simulink model "Model1_3_ZVD"  (R2021a)
settings: Solver=VariableStepAuto  StartTime=0.0  StopTime=20  RelTol=1e-3
InitFcn:
  | ml=2;
  | 
  | mc=0.5;
  | M2=0.5;
  | 
  | mt=5;
  | g=9.81;
  | l_ref=0.1;
  | l_ini=1;
  | l=l_ini;
  | x_ref=1;
  | n1=5;n2=1;
  | 
  | %ADRC' s parameter caculation
  | %b0 = (ml+mc)/(mc*ml +mc*mt+ml*mt); %Hieu
  | b0=(ml+mc)/(mt*mc+2*ml*mc+mt*ml+ml^2+mc^2); %Enhanced-coupling
  | k_ESO = 100;
  | T_set  = 6;
  | 
  | s_cl = -5.85/T_set;
  | Kp   = s_cl^2;
  | Kd   = -2*s_cl;
  | 
  | s_ESO = k_ESO*s_cl;
  | l1        = -3*s_ESO;
  | l2        = 3*( s_ESO)^2;
  | l3        = -(s_ESO)^3;
  | 
  | %b1 = (mt+mc)/(mc*ml +mc*mt+ml*mt);
  | b1=1/(ml+mc);
  | k_ESO1 =100;
  | T_set1  = 3;
  | s_cl1 = -5.85/T_set1;
  | Kp1   = s_cl1^2;
  | Kd1   = -2*s_cl1;
  | 
  | s_ESO1 = k_ESO1*s_cl1;
  | l11        = -3*s_ESO1;
  | l21        = 3*( s_ESO1)^2;
  | l31        = -(s_ESO1)^3;
  | 
  | 
  | L1=l_ini;
  | %L2=0.5;
  | L2=0.1;
  | m1=2;
  | m2=mc;
  | m=5;
  | %Bo input shaping
  | alpha = (1/L1 + 1/L2)*(m1+M2)/m1;
  | beta = (((m1+M2)/m1)^2)*((1/L1 + 1/L2)^2) - 4*(m1+M2)/(m1*L1*L2);
  | w1 = sqrt(g*(alpha - sqrt(beta))/2);
  | w2 = sqrt(g*(alpha + sqrt(beta))/2);
  | damping_ratio = 0;
  | wd1 = w1*sqrt(1-damping_ratio^2);
  | wd2 = w2*sqrt(1-damping_ratio^2);
  | k = exp(damping_ratio*pi/sqrt(1-damping_ratio^2));
  | 
  | %ZVD1
  | t1_ZVD_1=pi/wd1;
  | ... (+27 lines)
values from neighbouring files (symbols this model uses):
  particle = repmat(empty_particle, nPop, 1)    [PSO16_12.m]    (also in PSO_ZVD.m)
undefined symbols (not defined in the file or in its folder): E1_tt, E2_tt, E3_tt, i, li, xi
libraries: neural x66, simulink_extras x4, simulink x2
(part 12 of 20)

== matlab function Model1_3_ZVD/non linear model/con lắc đôi2/MATLAB Function ==
  data: z1 input; z2 input; z3 input; z4 input; z5 input; z6 input; z7 input; z8 input; d1z1 output; d1z2 output; d1z3 output; d1z4 output; d1z5 output; d1z6 output; d1z7 output; d1z8 output; ux input; ul input
function [d1z1,d1z2,d1z3,d1z4,d1z5,d1z6,d1z7,d1z8] = fcn(z1,z2, z3, z4, z5, z6, z7, z8, ux, ul)

m=20; m1=5; m2=1; l2= 0.2; g= 9.8;

d1z1=z2;
d1z2 =(m1*ul*sin(z5) - m2*ux - m1*ux + m2*ul*sin(z5) + m2*ux*cos(z5 - z7)^2 + m2*ux*sin(z5 - z7)^2 - m2*ul*sin(z5 - z7)*cos(z7) - g*m2^2*cos(z7)*sin(z7) - l2*m2^2*z8^2*sin(z7) - m2*ul*cos(z5 - z7)^2*sin(z5) + g*m2^2*cos(z5 - z7)*sin(z5 - z7)*cos(z5)^2 - g*m2^2*cos(z5 - z7)*sin(z5 - z7)*sin(z5)^2 + m2*ul*cos(z5 - z7)*sin(z5 - z7)*cos(z5) - g*m1*m2*cos(z7)*sin(z7) - l2*m1*m2*z8^2*sin(z7) + g*m2^2*cos(z5 - z7)*cos(z5)*sin(z7) + g*m2^2*cos(z5 - z7)*cos(z7)*sin(z5) - g*m2^2*sin(z5 - z7)*cos(z5)*cos(z7) + l2*m2^2*z8^2*cos(z5 - z7)*sin(z5) - l2*m2^2*z8^2*sin(z5 - z7)*cos(z5) + g*m2^2*sin(z5 - z7)*sin(z5)*sin(z7) - g*m2^2*cos(z5 - z7)^2*cos(z5)*sin(z5) - l2*m2^2*z8^2*cos(z5 - z7)^3*sin(z5) + l2*m2^2*z8^2*sin(z5 - z7)^3*cos(z5) + l2*m2^2*z8^2*cos(z5 - z7)^2*sin(z7) + g*m2^2*sin(z5 - z7)^2*cos(z5)*sin(z5) + l2*m2^2*z8^2*sin(z5 - z7)^2*sin(z7) + g*m1*m2*cos(z5 - z7)*sin(z5 - z7)*cos(z5)^2 - g*m1*m2*cos(z5 - z7)*sin(z5 - z7)*sin(z5)^2 + g*m1*m2*cos(z5 - z7)*cos(z5)*sin(z7) + g*m1*m2*cos(z5 - z7)*cos(z7)*sin(z5) - g*m1*m2*sin(z5 - z7)*cos(z5)*cos(z7) + l2*m1*m2*z8^2*cos(z5 - z7)*sin(z5) - l2*m1*m2*z8^2*sin(z5 - z7)*cos(z5) + g*m1*m2*sin(z5 - z7)*sin(z5)*sin(z7) - g*m1*m2*cos(z5 - z7)^2*cos(z5)*sin(z5) + l2*m2^2*z8^2*cos(z5 - z7)^2*sin(z5 - z7)*cos(z5) + g*m1*m2*sin(z5 - z7)^2*cos(z5)*sin(z5) - l2*m2^2*z8^2*cos(z5 - z7)*sin(z5 - z7)^2*sin(z5))/(m1^2*cos(z5)^2 - m*m2 - 2*m1*m2 - m*m1 + m2^2*cos(z5)^2 + m2^2*cos(z7)^2 + m1^2*sin(z5)^2 + m2^2*sin(z5)^2 + m2^2*cos(z5 - z7)^2 + m2^2*sin(z5 - z7)^2 - m1^2 - m2^2 + 2*m1*m2*cos(z5)^2 + m1*m2*cos(z7)^2 + 2*m1*m2*sin(z5)^2 + m*m2*cos(z5 - z7)^2 + m1*m2*cos(z5 - z7)^2 + m*m2*sin(z5 - z7)^2 + m1*m2*sin(z5 - z7)^2 - m2^2*cos(z5 - z7)^2*sin(z5)^2 - m2^2*sin(z5 - z7)^2*cos(z5)^2 - 2*m2^2*sin(z5 - z7)*cos(z7)*sin(z5) - m1*m2*cos(z5 - z7)^2*sin(z5)^2 - m1*m2*sin(z5 - z7)^2*cos(z5)^2 - 2*m2^2*cos(z5 - z7)*cos(z5)*cos(z7) - 2*m1*m2*cos(z5 - z7)*cos(z5)*cos(z7) - 2*m1*m2*sin(z5 - z7)*cos(z7)*sin(z5) + 2*m2^2*cos(z5 - z7)*sin(z5 - z7)*cos(z5)*sin(z5) + 2*m1*m2*cos(z5 - z7)*sin(z5 - z7)*cos(z5)*sin(z5));
d1z3=z4; 
d1z4 =(m2^2*ul*cos(z5 - z7)^2 - m2^2*ul - m1^2*ul - g*m1^3*cos(z5) - g*m2^3*cos(z5) - m1^3*z3*z6^2 - m2^3*z3*z6^2 + m1^2*ux*sin(z5) + m2^2*ux*sin(z5) - m*m1*ul - m*m2*ul - 2*m1*m2*ul + g*m1^3*cos(z5)^3 + g*m2^3*cos(z5)^3 + m1^2*ul*cos(z5)^2 + m2^2*ul*cos(z5)^2 + m2^2*ul*cos(z7)^2 - m2^2*ux*cos(z5 - z7)^2*sin(z5) + m2^3*z3*z6^2*sin(z5 - z7)^2 + m*m2*ul*cos(z5 - z7)^2 + m1*m2*ul*cos(z5 - z7)^2 + 3*g*m1*m2^2*cos(z5)^3 + 3*g*m1^2*m2*cos(z5)^3 - l2*m2^3*z8^2*cos(z5 - z7) + 2*m1*m2*ux*sin(z5) - m2^2*ux*sin(z5 - z7)*cos(z7) - g*m2^3*sin(z5 - z7)*sin(z7) + g*m2^3*cos(z5)*cos(z7)^2 + m1^3*z3*z6^2*cos(z5)^2 + m2^3*z3*z6^2*cos(z5)^2 + m2^3*z3*z6^2*cos(z7)^2 + g*m1^3*cos(z5)*sin(z5)^2 + g*m2^3*cos(z5)*sin(z5)^2 + m1^3*z3*z6^2*sin(z5)^2 + m2^3*z3*z6^2*sin(z5)^2 - g*m*m1^2*cos(z5) - g*m*m2^2*cos(z5) - 3*g*m1*m2^2*cos(z5) - 3*g*m1^2*m2*cos(z5) + g*m2^3*cos(z5 - z7)^2*cos(z5) + l2*m2^3*z8^2*cos(z5 - z7)^3 + 2*m1*m2*ul*cos(z5)^2 + m1*m2*ul*cos(z7)^2 - m*m1^2*z3*z6^2 - m*m2^2*z3*z6^2 - 3*m1*m2^2*z3*z6^2 - 3*m1^2*m2*z3*z6^2 + m2^3*z3*z6^2*cos(z5 - z7)^2 + l2*m2^3*z8^2*cos(z5 - z7)*sin(z5 - z7)^2 - m1*m2*ux*cos(z5 - z7)^2*sin(z5) - g*m*m2^2*sin(z5 - z7)*sin(z7) - 2*g*m1*m2^2*sin(z5 - z7)*sin(z7) - g*m1^2*m2*sin(z5 - z7)*sin(z7) + 2*g*m1*m2^2*cos(z5)*cos(z7)^2 + g*m1^2*m2*cos(z5)*cos(z7)^2 + 3*m1*m2^2*z3*z6^2*cos(z5)^2 + 3*m1^2*m2*z3*z6^2*cos(z5)^2 + 2*m1*m2^2*z3*z6^2*cos(z7)^2 + m1^2*m2*z3*z6^2*cos(z7)^2 + 3*g*m1*m2^2*cos(z5)*sin(z5)^2 + 3*g*m1^2*m2*cos(z5)*sin(z5)^2 + 3*m1*m2^2*z3*z6^2*sin(z5)^2 + 3*m1^2*m2*z3*z6^2*sin(z5)^2 - m2^3*z3*z6^2*cos(z5 - z7)^2*sin(z5)^2 - m2^3*z3*z6^2*sin(z5 - z7)^2*cos(z5)^2 + g*m2^3*cos(z7)*sin(z5)*sin(z7) + l2*m2^3*z8^2*sin(z5)*sin(z7) + g*m*m2^2*cos(z5 - z7)^2*cos(z5) + 2*g*m1*m2^2*cos(z5 - z7)^2*cos(z5) + g*m1^2*m2*cos(z5 - z7)^2*cos(z5) + l2*m*m2^2*z8^2*cos(z5 - z7)^3 + l2*m1*m2^2*z8^2*cos(z5 - z7)^3 + m*m2^2*z3*z6^2*cos(z5 - z7)^2 + 2*m1*m2^2*z3*z6^2*cos(z5 - z7)^2 + m1^2*m2*z3*z6^2*cos(z5 - z7)^2 + m*m2^2*z3*z6^2*sin(z5 - z7)^2 + 2*m1*m2^2*z3*z6^2*sin(z5 - z7)^2 + m1^2*m2*z3*z6^2*sin(z5 - z7)^2 - 2*m2^2*ul*cos(z5 - z7)*cos(z5)*cos(z7) - m1*m2*ux*sin(z5 - z7)*cos(z7) + m2^2*ux*cos(z5 - z7)*sin(z5 - z7)*cos(z5) + g*m2^3*cos(z5 - z7)*sin(z5 - z7)*sin(z5) - 2*g*m2^3*cos(z5 - z7)*cos(z5)^2*cos(z7) + l2*m2^3*z8^2*cos(z5 - z7)*cos(z5)^2 + l2*m2^3*z8^2*cos(z5 - z7)*cos(z7)^2 - g*m2^3*cos(z5 - z7)*cos(z7)*sin(z5)^2 + g*m2^3*sin(z5 - z7)*cos(z5)^2*sin(z7) - 2*g*m*m1*m2*cos(z5) - l2*m*m2^2*z8^2*cos(z5 - z7) - 2*l2*m1*m2^2*z8^2*cos(z5 - z7) - l2*m1^2*m2*z8^2*cos(z5 - z7) - 2*m*m1*m2*z3*z6^2 - l2*m*m1*m2*z8^2*cos(z5 - z7) - g*m*m1*m2*sin(z5 - z7)*sin(z7) + g*m*m2^2*cos(z5 - z7)*sin(z5 - z7)*sin(z5) + 2*g*m1*m2^2*cos(z5 - z7)*sin(z5 - z7)*sin(z5) + g*m1^2*m2*cos(z5 - z7)*sin(z5 - z7)*sin(z5) - 4*g*m1*m2^2*cos(z5 - z7)*cos(z5)^2*cos(z7) - 2*g*m1^2*m2*cos(z5 - z7)*cos(z5)^2*cos(z7) + 2*l2*m1*m2^2*z8^2*cos(z5 - z7)*cos(z5)^2 + l2*m1^2*m2*z8^2*cos(z5 - z7)*cos(z5)^2 + l2*m1*m2^2*z8^2*cos(z5 - z7)*cos(z7)^2 - 2*g*m1*m2^2*cos(z5 - z7)*cos(z7)*sin(z5)^2 - g*m1^2*m2*cos(z5 - z7)*cos(z7)*sin(z5)^2 + 2*g*m1*m2^2*sin(z5 - z7)*cos(z5)^2*sin(z7) + g*m1^2*m2*sin(z5 - z7)*cos(z5)^2*sin(z7) - 2*m2^3*z3*z6^2*cos(z5 - z7)*cos(z5)*cos(z7) + g*m*m1*m2*cos(z5 - z7)^2*cos(z5) - g*m2^3*cos(z5 - z7)*cos(z5)*sin(z5)*sin(z7) - g*m2^3*sin(z5 - z7)*cos(z5)*cos(z7)*sin(z5) + l2*m2^3*z8^2*sin(z5 - z7)*cos(z5)*sin(z5) - l2*m2^3*z8^2*sin(z5 - z7)*cos(z7)*sin(z7) + m*m1*m2*z3*z6^2*cos(z5 - z7)^2 - 2*m2^3*z3*z6^2*sin(z5 - z7)*cos(z7)*sin(z5) + l2*m*m2^2*z8^2*cos(z5 - z7)*sin(z5 - z7)^2 + l2*m1*m2^2*z8^2*cos(z5 - z7)*sin(z5 - z7)^2 + m*m1*m2*z3*z6^2*sin(z5 - z7)^2 - 2*m1*m2*ul*cos(z5 - z7)*cos(z5)*cos(z7) - 2*l2*m2^3*z8^2*cos(z5 - z7)^2*cos(z5)*cos(z7) - 2*m1*m2^2*z3*z6^2*cos(z5 - z7)^2*sin(z5)^2 - 2*m1*m2^2*z3*z6^2*sin(z5 - z7)^2*cos(z5)^2 - m1^2*m2*z3*z6^2*cos(z5 - z7)^2*sin(z5)^2 - m1^2*m2*z3*z6^2*sin(z5 - z7)^2*cos(z5)^2 - l2*m2^3*z8^2*sin(z5 - z7)^2*cos(z5)*cos(z7) + 2*g*m1*m2^2*cos(z7)*sin(z5)*sin(z7) + g*m1^2*m2*cos(z7)*sin(z5)*sin(z7) + 2*l2*m1*m2^2*z8^2*sin(z5)*sin(z7) + l2*m1^2*m2*z8^2*sin(z5)*sin(z7) - l2*m2^3*z8^2*cos(z5 - z7)^2*sin(z5)*sin(z7) + m1*m2*ux*cos(z5 - z7)*sin(z5 - z7)*cos(z5) - 2*l2*m1*m2^2*z8^2*cos(z5 - z7)^2*cos(z5)*cos(z7) - l2*m1*m2^2*z8^2*sin(z5 - z7)^2*cos(z5)*cos(z7) - l2*m1*m2^2*z8^2*cos(z5 - z7)^2*sin(z5)*sin(z7) + g*m*m1*m2*cos(z5 - z7)*sin(z5 - z7)*sin(z5) + l2*m2^3*z8^2*cos(z5 - z7)*sin(z5 - z7)*cos(z5)*sin(z7) - l2*m2^3*z8^2*cos(z5 - z7)*sin(z5 - z7)*cos(z7)*sin(z5) + 2*m2^3*z3*z6^2*cos(z5 - z7)*sin(z5 - z7)*cos(z5)*sin(z5) - 4*m1*m2^2*z3*z6^2*cos(z5 - z7)*cos(z5)*cos(z7) - 2*m1^2*m2*z3*z6^2*cos(z5 - z7)*cos(z5)*cos(z7) - 2*g*m1*m2^2*cos(z5 - z7)*cos(z5)*sin(z5)*sin(z7) - 2*g*m1*m2^2*sin(z5 - z7)*cos(z5)*cos(z7)*sin(z5) - g*m1^2*m2*cos(z5 - z7)*cos(z5)*sin(z5)*sin(z7) - g*m1^2*m2*sin(z5 - z7)*cos(z5)*cos(z7)*sin(z5) + 2*l2*m1*m2^2*z8^2*sin(z5 - z7)*cos(z5)*sin(z5) + l2*m1^2*m2*z8^2*sin(z5 - z7)*cos(z5)*sin(z5) - l2*m1*m2^2*z8^2*sin(z5 - z7)*cos(z7)*sin(z7) - 4*m1*m2^2*z3*z6^2*sin(z5 - z7)*cos(z7)*sin(z5) - 2*m1^2*m2*z3*z6^2*sin(z5 - z7)*cos(z7)*sin(z5) + l2*m1*m2^2*z8^2*cos(z5 - z7)*sin(z5 - z7)*cos(z5)*sin(z7) - l2*m1*m2^2*z8^2*cos(z5 - z7)*sin(z5 - z7)*cos(z7)*sin(z5) + 4*m1*m2^2*z3*z6^2*cos(z5 - z7)*sin(z5 - z7)*cos(z5)*sin(z5) + 2*m1^2*m2*z3*z6^2*cos(z5 - z7)*sin(z5 - z7)*cos(z5)*sin(z5))/((m1 + m2)*(m1^2*cos(z5)^2 - m*m2 - 2*m1*m2 - m*m1 + m2^2*cos(z5)^2 + m2^2*cos(z7)^2 + m1^2*sin(z5)^2 + m2^2*sin(z5)^2 + m2^2*cos(z5 - z7)^2 + m2^2*sin(z5 - z7)^2 - m1^2 - m2^2 + 2*m1*m2*cos(z5)^2 + m1*m2*cos(z7)^2 + 2*m1*m2*sin(z5)^2 + m*m2*cos(z5 - z7)^2 + m1*m2*cos(z5 - z7)^2 + m*m2*sin(z5 - z7)^2 + m1*m2*sin(z5 - z7)^2 - m2^2*cos(z5 - z7)^2*sin(z5)^2 - m2^2*sin(z5 - z7)^2*cos(z5)^2 - 2*m2^2*sin(z5 - z7)*cos(z7)*sin(z5) - m1*m2*cos(z5 - z7)^2*sin(z5)^2 - m1*m2*sin(z5 - z7)^2*cos(z5)^2 - 2*m2^2*cos(z5 - z7)*cos(z5)*cos(z7) - 2*m1*m2*cos(z5 - z7)*cos(z5)*cos(z7) - 2*m1*m2*sin(z5 - z7)*cos(z7)*sin(z5) + 2*m2^2*cos(z5 - z7)*sin(z5 - z7)*cos(z5)*sin(z5) + 2*m1*m2*cos(z5 - z7)*sin(z5 - z7)*cos(z5)*sin(z5)));
d1z5=z6; 
d1z6 =-(g*m1^3*sin(z5)^3 - 2*m2^3*z4*z6 - m1^2*ux*cos(z5) - m2^2*ux*cos(z5) - g*m1^3*sin(z5) - g*m2^3*sin(z5) - 2*m1^3*z4*z6 + g*m2^3*sin(z5)^3 + m2^2*ux*sin(z5 - z7)^2*cos(z5) + g*m2^3*sin(z5 - z7)^2*sin(z5) + 3*g*m1*m2^2*sin(z5)^3 + 3*g*m1^2*m2*sin(z5)^3 + 2*m1^3*z4*z6*cos(z5)^2 + 2*m2^3*z4*z6*cos(z5)^2 + 2*m2^3*z4*z6*cos(z7)^2 + m1^2*ul*cos(z5)*sin(z5) + m2^2*ul*cos(z5)*sin(z5) + 2*m1^3*z4*z6*sin(z5)^2 + 2*m2^3*z4*z6*sin(z5)^2 - 2*m1*m2*ux*cos(z5) - 2*m*m1^2*z4*z6 - 2*m*m2^2*z4*z6 - 6*m1*m2^2*z4*z6 - 6*m1^2*m2*z4*z6 + m2^2*ux*cos(z5 - z7)*cos(z7) + 2*m2^3*z4*z6*cos(z5 - z7)^2 + g*m2^3*cos(z5 - z7)*sin(z7) - l2*m2^3*z8^2*sin(z5 - z7) + 2*m2^3*z4*z6*sin(z5 - z7)^2 + g*m1^3*cos(z5)^2*sin(z5) + g*m2^3*cos(z5)^2*sin(z5) + g*m2^3*cos(z7)^2*sin(z5) + m2^2*ul*cos(z5 - z7)*sin(z5 - z7) - g*m*m1^2*sin(z5) - g*m*m2^2*sin(z5) - 3*g*m1*m2^2*sin(z5) - 3*g*m1^2*m2*sin(z5) + l2*m2^3*z8^2*sin(z5 - z7)^3 + 2*m*m2^2*z4*z6*cos(z5 - z7)^2 + 4*m1*m2^2*z4*z6*cos(z5 - z7)^2 + 2*m1^2*m2*z4*z6*cos(z5 - z7)^2 + g*m*m2^2*cos(z5 - z7)*sin(z7) + 2*g*m1*m2^2*cos(z5 - z7)*sin(z7) + g*m1^2*m2*cos(z5 - z7)*sin(z7) - l2*m*m2^2*z8^2*sin(z5 - z7) - 2*l2*m1*m2^2*z8^2*sin(z5 - z7) - l2*m1^2*m2*z8^2*sin(z5 - z7) + l2*m2^3*z8^2*cos(z5 - z7)^2*sin(z5 - z7) + m1*m2*ux*sin(z5 - z7)^2*cos(z5) + 2*m*m2^2*z4*z6*sin(z5 - z7)^2 + 4*m1*m2^2*z4*z6*sin(z5 - z7)^2 + 2*m1^2*m2*z4*z6*sin(z5 - z7)^2 + 3*g*m1*m2^2*cos(z5)^2*sin(z5) + 3*g*m1^2*m2*cos(z5)^2*sin(z5) + 2*g*m1*m2^2*cos(z7)^2*sin(z5) + g*m1^2*m2*cos(z7)^2*sin(z5) - g*m2^3*cos(z5)*cos(z7)*sin(z7) - l2*m2^3*z8^2*cos(z5)*sin(z7) + l2*m*m2^2*z8^2*sin(z5 - z7)^3 + l2*m1*m2^2*z8^2*sin(z5 - z7)^3 + g*m*m2^2*sin(z5 - z7)^2*sin(z5) + 2*g*m1*m2^2*sin(z5 - z7)^2*sin(z5) + g*m1^2*m2*sin(z5 - z7)^2*sin(z5) + 2*m1*m2*ul*cos(z5)*sin(z5) - m2^2*ul*cos(z5 - z7)*cos(z7)*sin(z5) - m2^2*ul*sin(z5 - z7)*cos(z5)*cos(z7) - 4*m*m1*m2*z4*z6 + m1*m2*ux*cos(z5 - z7)*cos(z7) + g*m2^3*cos(z5 - z7)*sin(z5 - z7)*cos(z5) + 6*m1*m2^2*z4*z6*cos(z5)^2 + 6*m1^2*m2*z4*z6*cos(z5)^2 + 4*m1*m2^2*z4*z6*cos(z7)^2 + 2*m1^2*m2*z4*z6*cos(z7)^2 - m2^2*ux*cos(z5 - z7)*sin(z5 - z7)*sin(z5) - g*m2^3*sin(z5 - z7)*cos(z5)^2*cos(z7) + l2*m2^3*z8^2*sin(z5 - z7)*cos(z7)^2 + 6*m1*m2^2*z4*z6*sin(z5)^2 + 6*m1^2*m2*z4*z6*sin(z5)^2 - 2*m2^3*z4*z6*cos(z5 - z7)^2*sin(z5)^2 - 2*m2^3*z4*z6*sin(z5 - z7)^2*cos(z5)^2 - g*m2^3*cos(z5 - z7)*sin(z5)^2*sin(z7) - 2*g*m2^3*sin(z5 - z7)*cos(z7)*sin(z5)^2 + l2*m2^3*z8^2*sin(z5 - z7)*sin(z5)^2 + m*m2*ul*cos(z5 - z7)*sin(z5 - z7) + m1*m2*ul*cos(z5 - z7)*sin(z5 - z7) - 2*g*m*m1*m2*sin(z5) + 2*m*m1*m2*z4*z6*cos(z5 - z7)^2 - 4*m2^3*z4*z6*sin(z5 - z7)*cos(z7)*sin(z5) + g*m*m1*m2*cos(z5 - z7)*sin(z7) - l2*m*m1*m2*z8^2*sin(z5 - z7) + g*m*m2^2*cos(z5 - z7)*sin(z5 - z7)*cos(z5) + 2*g*m1*m2^2*cos(z5 - z7)*sin(z5 - z7)*cos(z5) + g*m1^2*m2*cos(z5 - z7)*sin(z5 - z7)*cos(z5) + 2*m*m1*m2*z4*z6*sin(z5 - z7)^2 - 2*g*m1*m2^2*sin(z5 - z7)*cos(z5)^2*cos(z7) - g*m1^2*m2*sin(z5 - z7)*cos(z5)^2*cos(z7) + l2*m1*m2^2*z8^2*sin(z5 - z7)*cos(z7)^2 - 4*m1*m2^2*z4*z6*cos(z5 - z7)^2*sin(z5)^2 - 4*m1*m2^2*z4*z6*sin(z5 - z7)^2*cos(z5)^2 - 2*m1^2*m2*z4*z6*cos(z5 - z7)^2*sin(z5)^2 - 2*m1^2*m2*z4*z6*sin(z5 - z7)^2*cos(z5)^2 - 2*g*m1*m2^2*cos(z5 - z7)*sin(z5)^2*sin(z7) - 4*g*m1*m2^2*sin(z5 - z7)*cos(z7)*sin(z5)^2 - g*m1^2*m2*cos(z5 - z7)*sin(z5)^2*sin(z7) - 2*g*m1^2*m2*sin(z5 - z7)*cos(z7)*sin(z5)^2 + 2*l2*m1*m2^2*z8^2*sin(z5 - z7)*sin(z5)^2 + l2*m1^2*m2*z8^2*sin(z5 - z7)*sin(z5)^2 - g*m2^3*cos(z5 - z7)*cos(z5)*cos(z7)*sin(z5) + l2*m2^3*z8^2*cos(z5 - z7)*cos(z5)*sin(z5) + l2*m2^3*z8^2*cos(z5 - z7)*cos(z7)*sin(z7) + g*m2^3*sin(z5 - z7)*cos(z5)*sin(z5)*sin(z7) + l2*m*m2^2*z8^2*cos(z5 - z7)^2*sin(z5 - z7) + l2*m1*m2^2*z8^2*cos(z5 - z7)^2*sin(z5 - z7) + g*m*m1*m2*sin(z5 - z7)^2*sin(z5) - m1*m2*ul*cos(z5 - z7)*cos(z7)*sin(z5) - m1*m2*ul*sin(z5 - z7)*cos(z5)*cos(z7) - 2*g*m1*m2^2*cos(z5)*cos(z7)*sin(z7) - g*m1^2*m2*cos(z5)*cos(z7)*sin(z7) - 2*l2*m1*m2^2*z8^2*cos(z5)*sin(z7) - l2*m1^2*m2*z8^2*cos(z5)*sin(z7) - l2*m2^3*z8^2*cos(z5 - z7)^2*cos(z7)*sin(z5) + l2*m2^3*z8^2*sin(z5 - z7)^2*cos(z5)*sin(z7) - 2*l2*m2^3*z8^2*sin(z5 - z7)^2*cos(z7)*sin(z5) - m1*m2*ux*cos(z5 - z7)*sin(z5 - z7)*sin(z5) - 4*m2^3*z4*z6*cos(z5 - z7)*cos(z5)*cos(z7) - l2*m1*m2^2*z8^2*cos(z5 - z7)^2*cos(z7)*sin(z5) + 4*m2^3*z4*z6*cos(z5 - z7)*sin(z5 - z7)*cos(z5)*sin(z5) + g*m*m1*m2*cos(z5 - z7)*sin(z5 - z7)*cos(z5) + l2*m1*m2^2*z8^2*sin(z5 - z7)^2*cos(z5)*sin(z7) - 2*l2*m1*m2^2*z8^2*sin(z5 - z7)^2*cos(z7)*sin(z5) - 8*m1*m2^2*z4*z6*cos(z5 - z7)*cos(z5)*cos(z7) - 4*m1^2*m2*z4*z6*cos(z5 - z7)*cos(z5)*cos(z7) - l2*m2^3*z8^2*cos(z5 - z7)*sin(z5 - z7)*cos(z5)*cos(z7) - 8*m1*m2^2*z4*z6*sin(z5 - z7)*cos(z7)*sin(z5) - 4*m1^2*m2*z4*z6*sin(z5 - z7)*cos(z7)*sin(z5) - l2*m2^3*z8^2*cos(z5 - z7)*sin(z5 - z7)*sin(z5)*sin(z7) - 2*g*m1*m2^2*cos(z5 - z7)*cos(z5)*cos(z7)*sin(z5) - g*m1^2*m2*cos(z5 - z7)*cos(z5)*cos(z7)*sin(z5) + 2*l2*m1*m2^2*z8^2*cos(z5 - z7)*cos(z5)*sin(z5) + l2*m1^2*m2*z8^2*cos(z5 - z7)*cos(z5)*sin(z5) + l2*m1*m2^2*z8^2*cos(z5 - z7)*cos(z7)*sin(z7) + 2*g*m1*m2^2*sin(z5 - z7)*cos(z5)*sin(z5)*sin(z7) + g*m1^2*m2*sin(z5 - z7)*cos(z5)*sin(z5)*sin(z7) + 8*m1*m2^2*z4*z6*cos(z5 - z7)*sin(z5 - z7)*cos(z5)*sin(z5) + 4*m1^2*m2*z4*z6*cos(z5 - z7)*sin(z5 - z7)*cos(z5)*sin(z5) - l2*m1*m2^2*z8^2*cos(z5 - z7)*sin(z5 - z7)*cos(z5)*cos(z7) - l2*m1*m2^2*z8^2*cos(z5 - z7)*sin(z5 - z7)*sin(z5)*sin(z7))/(z3*(m1 + m2)*(m1^2*cos(z5)^2 - m*m2 - 2*m1*m2 - m*m1 + m2^2*cos(z5)^2 + m2^2*cos(z7)^2 + m1^2*sin(z5)^2 + m2^2*sin(z5)^2 + m2^2*cos(z5 - z7)^2 + m2^2*sin(z5 - z7)^2 - m1^2 - m2^2 + 2*m1*m2*cos(z5)^2 + m1*m2*cos(z7)^2 + 2*m1*m2*sin(z5)^2 + m*m2*cos(z5 - z7)^2 + m1*m2*cos(z5 - z7)^2 + m*m2*sin(z5 - z7)^2 + m1*m2*sin(z5 - z7)^2 - m2^2*cos(z5 - z7)^2*sin(z5)^2 - m2^2*sin(z5 - z7)^2*cos(z5)^2 - 2*m2^2*sin(z5 - z7)*cos(z7)*sin(z5) - m1*m2*cos(z5 - z7)^2*sin(z5)^2 - m1*m2*sin(z5 - z7)^2*cos(z5)^2 - 2*m2^2*cos(z5 - z7)*cos(z5)*cos(z7) - 2*m1*m2*cos(z5 - z7)*cos(z5)*cos(z7) - 2*m1*m2*sin(z5 - z7)*cos(z7)*sin(z5) + 2*m2^2*cos(z5 - z7)*sin(z5 - z7)*cos(z5)*sin(z5) + 2*m1*m2*cos(z5 - z7)*sin(z5 - z7)*cos(z5)*sin(z5)));
d1z7 = z8;
d1z8 =-(m1*ul*cos(z7)*sin(z5) - m2*ux*cos(z7) - m*ul*sin(z5 - z7) - m1*ul*sin(z5 - z7) - m2*ul*sin(z5 - z7) - g*m1^2*sin(z7) - g*m2^2*sin(z7) - m1*ux*cos(z7) + m2*ul*cos(z7)*sin(z5) + m1*ux*cos(z5 - z7)*cos(z5) + m2*ux*cos(z5 - z7)*cos(z5) + m1*ux*sin(z5 - z7)*sin(z5) + m2*ux*sin(z5 - z7)*sin(z5) - g*m*m1*sin(z7) - g*m*m2*sin(z7) - 2*g*m1*m2*sin(z7) + g*m1^2*cos(z5 - z7)*sin(z5) - g*m1^2*sin(z5 - z7)*cos(z5) + g*m2^2*cos(z5 - z7)*sin(z5) - g*m2^2*sin(z5 - z7)*cos(z5) + m1*ul*sin(z5 - z7)*cos(z5)^2 + m2*ul*sin(z5 - z7)*cos(z5)^2 + g*m1^2*cos(z5)^2*sin(z7) + g*m2^2*cos(z5)^2*sin(z7) + g*m1^2*sin(z5)^2*sin(z7) + g*m2^2*sin(z5)^2*sin(z7) - g*m1^2*cos(z5 - z7)*sin(z5)^3 + g*m1^2*sin(z5 - z7)*cos(z5)^3 - g*m2^2*cos(z5 - z7)*sin(z5)^3 + g*m2^2*sin(z5 - z7)*cos(z5)^3 - 2*g*m1*m2*cos(z5 - z7)*sin(z5)^3 + 2*g*m1*m2*sin(z5 - z7)*cos(z5)^3 - m1*ul*cos(z5 - z7)*cos(z5)*sin(z5) - m2*ul*cos(z5 - z7)*cos(z5)*sin(z5) - l2*m2^2*z8^2*cos(z7)*sin(z7) + g*m*m1*cos(z5 - z7)*sin(z5) - g*m*m1*sin(z5 - z7)*cos(z5) + g*m*m2*cos(z5 - z7)*sin(z5) - g*m*m2*sin(z5 - z7)*cos(z5) + 2*g*m1*m2*cos(z5 - z7)*sin(z5) - 2*g*m1*m2*sin(z5 - z7)*cos(z5) + 2*g*m1*m2*cos(z5)^2*sin(z7) - g*m1^2*cos(z5 - z7)*cos(z5)^2*sin(z5) - g*m2^2*cos(z5 - z7)*cos(z5)^2*sin(z5) + 2*g*m1*m2*sin(z5)^2*sin(z7) + g*m1^2*sin(z5 - z7)*cos(z5)*sin(z5)^2 + g*m2^2*sin(z5 - z7)*cos(z5)*sin(z5)^2 - l2*m1*m2*z8^2*cos(z7)*sin(z7) + l2*m2^2*z8^2*cos(z5 - z7)*cos(z5)*sin(z7) + l2*m2^2*z8^2*cos(z5 - z7)*cos(z7)*sin(z5) - l2*m2^2*z8^2*sin(z5 - z7)*cos(z5)*cos(z7) + l2*m2^2*z8^2*sin(z5 - z7)*sin(z5)*sin(z7) - l2*m2^2*z8^2*cos(z5 - z7)^2*cos(z5)*sin(z5) + l2*m2^2*z8^2*sin(z5 - z7)^2*cos(z5)*sin(z5) - 2*g*m1*m2*cos(z5 - z7)*cos(z5)^2*sin(z5) + l2*m2^2*z8^2*cos(z5 - z7)*sin(z5 - z7)*cos(z5)^2 + 2*g*m1*m2*sin(z5 - z7)*cos(z5)*sin(z5)^2 - l2*m2^2*z8^2*cos(z5 - z7)*sin(z5 - z7)*sin(z5)^2 - l2*m1*m2*z8^2*cos(z5 - z7)*sin(z5 - z7)*sin(z5)^2 + l2*m1*m2*z8^2*cos(z5 - z7)*cos(z5)*sin(z7) + l2*m1*m2*z8^2*cos(z5 - z7)*cos(z7)*sin(z5) - l2*m1*m2*z8^2*sin(z5 - z7)*cos(z5)*cos(z7) + l2*m1*m2*z8^2*sin(z5 - z7)*sin(z5)*sin(z7) - l2*m1*m2*z8^2*cos(z5 - z7)^2*cos(z5)*sin(z5) + l2*m1*m2*z8^2*sin(z5 - z7)^2*cos(z5)*sin(z5) + l2*m1*m2*z8^2*cos(z5 - z7)*sin(z5 - z7)*cos(z5)^2)/(l2*(m1^2*cos(z5)^2 - m*m2 - 2*m1*m2 - m*m1 + m2^2*cos(z5)^2 + m2^2*cos(z7)^2 + m1^2*sin(z5)^2 + m2^2*sin(z5)^2 + m2^2*cos(z5 - z7)^2 + m2^2*sin(z5 - z7)^2 - m1^2 - m2^2 + 2*m1*m2*cos(z5)^2 + m1*m2*cos(z7)^2 + 2*m1*m2*sin(z5)^2 + m*m2*cos(z5 - z7)^2 + m1*m2*cos(z5 - z7)^2 + m*m2*sin(z5 - z7)^2 + m1*m2*sin(z5 - z7)^2 - m2^2*cos(z5 - z7)^2*sin(z5)^2 - m2^2*sin(z5 - z7)^2*cos(z5)^2 - 2*m2^2*sin(z5 - z7)*cos(z7)*sin(z5) - m1*m2*cos(z5 - z7)^2*sin(z5)^2 - m1*m2*sin(z5 - z7)^2*cos(z5)^2 - 2*m2^2*cos(z5 - z7)*cos(z5)*cos(z7) - 2*m1*m2*cos(z5 - z7)*cos(z5)*cos(z7) - 2*m1*m2*sin(z5 - z7)*cos(z7)*sin(z5) + 2*m2^2*cos(z5 - z7)*sin(z5 - z7)*cos(z5)*sin(z5) + 2*m1*m2*cos(z5 - z7)*sin(z5 - z7)*cos(z5)*sin(z5)));

== matlab function Model1_3_ZVD/RBF_ZVD_m=5_m1=1/enhanced1/Crane ==
  data: dx1 output; d1x input; l1 input; d1l1 input; the1 input; d1the1 input; the2 input; d1the2 input; Fx input; Fl input; dx2 output; dx3 output; dx4 output; dx5 output; dx6 output; m2 input; dx7 output; dx8 output
function [dx1,dx2,dx3,dx4,dx5,dx6,dx7,dx8] = fcn(d1x,l1,d1l1,the1,d1the1,the2,d1the2,Fx,Fl,m2)
 m =5; m1 =2; g =9.81; l2=0.5;bx=25; bl=50;bc=0.1;

 dx1=d1x;

 dx2 = (Fx*l1*l2*m2*cos(the1 - the2)^2 - Fx*l1*l2*m2 - d1the2^2*l1*l2^2*m2^2*sin(the2) - Fx*l1*l2*m1 + Fx*l1*l2*m2*sin(the1 - the2)^2 + bx*d1x*l1*l2*m1 + bx*d1x*l1*l2*m2 + Fl*l1*l2*m1*sin(the1) + Fl*l1*l2*m2*sin(the1) - bc*d1the1*l2*m1*cos(the1) - bc*d1the1*l2*m2*cos(the1) - bc*d1the2*l1*m1*cos(the2) - bc*d1the2*l1*m2*cos(the2) + bc*d1the2*l1*m1*sin(the1 - the2)*sin(the1) + bc*d1the2*l1*m2*sin(the1 - the2)*sin(the1) + d1the2^2*l1*l2^2*m2^2*cos(the1 - the2)*sin(the1) - d1the2^2*l1*l2^2*m2^2*sin(the1 - the2)*cos(the1) - d1the2^2*l1*l2^2*m1*m2*sin(the2) - g*l1*l2*m2^2*cos(the2)*sin(the2) - Fl*l1*l2*m2*cos(the1 - the2)^2*sin(the1) + bc*d1the1*l2*m2*sin(the1 - the2)^2*cos(the1) - bl*d1l1*l1*l2*m1*sin(the1) - bl*d1l1*l1*l2*m2*sin(the1) + d1the2^2*l1*l2^2*m2^2*cos(the1 - the2)^2*sin(the2) - d1the2^2*l1*l2^2*m2^2*cos(the1 - the2)^3*sin(the1) + d1the2^2*l1*l2^2*m2^2*sin(the1 - the2)^3*cos(the1) + d1the2^2*l1*l2^2*m2^2*sin(the1 - the2)^2*sin(the2) - bx*d1x*l1*l2*m2*cos(the1 - the2)^2 - Fl*l1*l2*m2*sin(the1 - the2)*cos(the2) + bc*d1the2*l1*m1*cos(the1 - the2)*cos(the1) + bc*d1the2*l1*m2*cos(the1 - the2)*cos(the1) + bc*d1the1*l2*m2*cos(the1 - the2)*cos(the2) - bx*d1x*l1*l2*m2*sin(the1 - the2)^2 - bc*d1the1*l2*m2*cos(the1 - the2)*sin(the1 - the2)*sin(the1) + d1the2^2*l1*l2^2*m1*m2*cos(the1 - the2)*sin(the1) - d1the2^2*l1*l2^2*m1*m2*sin(the1 - the2)*cos(the1) + g*l1*l2*m2^2*cos(the1 - the2)*cos(the1)*sin(the2) + g*l1*l2*m2^2*cos(the1 - the2)*cos(the2)*sin(the1) - g*l1*l2*m2^2*sin(the1 - the2)*cos(the1)*cos(the2) - g*l1*l2*m1*m2*cos(the2)*sin(the2) + g*l1*l2*m2^2*sin(the1 - the2)*sin(the1)*sin(the2) + bl*d1l1*l1*l2*m2*sin(the1 - the2)*cos(the2) + d1the2^2*l1*l2^2*m2^2*cos(the1 - the2)^2*sin(the1 - the2)*cos(the1) - d1the2^2*l1*l2^2*m2^2*cos(the1 - the2)*sin(the1 - the2)^2*sin(the1) - g*l1*l2*m2^2*cos(the1 - the2)^2*cos(the1)*sin(the1) + g*l1*l2*m2^2*sin(the1 - the2)^2*cos(the1)*sin(the1) + bl*d1l1*l1*l2*m2*cos(the1 - the2)^2*sin(the1) + g*l1*l2*m2^2*cos(the1 - the2)*sin(the1 - the2)*cos(the1)^2 - g*l1*l2*m2^2*cos(the1 - the2)*sin(the1 - the2)*sin(the1)^2 + Fl*l1*l2*m2*cos(the1 - the2)*sin(the1 - the2)*cos(the1) + g*l1*l2*m1*m2*cos(the1 - the2)*cos(the1)*sin(the2) + g*l1*l2*m1*m2*cos(the1 - the2)*cos(the2)*sin(the1) - g*l1*l2*m1*m2*sin(the1 - the2)*cos(the1)*cos(the2) + g*l1*l2*m1*m2*sin(the1 - the2)*sin(the1)*sin(the2) - bl*d1l1*l1*l2*m2*cos(the1 - the2)*sin(the1 - the2)*cos(the1) - g*l1*l2*m1*m2*cos(the1 - the2)^2*cos(the1)*sin(the1) + g*l1*l2*m1*m2*sin(the1 - the2)^2*cos(the1)*sin(the1) + g*l1*l2*m1*m2*cos(the1 - the2)*sin(the1 - the2)*cos(the1)^2 - g*l1*l2*m1*m2*cos(the1 - the2)*sin(the1 - the2)*sin(the1)^2)/(l1*l2*(m1^2*cos(the1)^2 - m*m2 - 2*m1*m2 - m*m1 + m2^2*cos(the1)^2 + m2^2*cos(the2)^2 + m1^2*sin(the1)^2 + m2^2*sin(the1)^2 + m2^2*cos(the1 - the2)^2 + m2^2*sin(the1 - the2)^2 - m1^2 - m2^2 + 2*m1*m2*cos(the1)^2 + m1*m2*cos(the2)^2 + 2*m1*m2*sin(the1)^2 + m*m2*cos(the1 - the2)^2 + m1*m2*cos(the1 - the2)^2 + m*m2*sin(the1 - the2)^2 + m1*m2*sin(the1 - the2)^2 - m2^2*cos(the1 - the2)^2*sin(the1)^2 - m2^2*sin(the1 - the2)^2*cos(the1)^2 - 2*m2^2*sin(the1 - the2)*cos(the2)*sin(the1) - 2*m2^2*cos(the1 - the2)*cos(the1)*cos(the2) - m1*m2*cos(the1 - the2)^2*sin(the1)^2 - m1*m2*sin(the1 - the2)^2*cos(the1)^2 + 2*m2^2*cos(the1 - the2)*sin(the1 - the2)*cos(the1)*sin(the1) - 2*m1*m2*sin(the1 - the2)*cos(the2)*sin(the1) - 2*m1*m2*cos(the1 - the2)*cos(the1)*cos(the2) + 2*m1*m2*cos(the1 - the2)*sin(the1 - the2)*cos(the1)*sin(the1)));

 dx3=d1l1;

 dx4 = (Fx*l1*l2*m1^2*sin(the1) - d1the1^2*l1^2*l2*m2^3 - Fl*l1*l2*m1^2 - Fl*l1*l2*m2^2 - d1the2^2*l1*l2^2*m2^3*cos(the1 - the2) - d1the1^2*l1^2*l2*m1^3 + Fx*l1*l2*m2^2*sin(the1) - g*l1*l2*m1^3*cos(the1) - g*l1*l2*m2^3*cos(the1) - Fl*l1*l2*m*m1 - Fl*l1*l2*m*m2 - 2*Fl*l1*l2*m1*m2 + d1the1^2*l1^2*l2*m1^3*cos(the1)^2 + d1the1^2*l1^2*l2*m2^3*cos(the1)^2 + d1the1^2*l1^2*l2*m2^3*cos(the2)^2 + d1the1^2*l1^2*l2*m1^3*sin(the1)^2 + d1the1^2*l1^2*l2*m2^3*sin(the1)^2 - bc*d1the2*l1*m1^2*sin(the1 - the2) - bc*d1the2*l1*m2^2*sin(the1 - the2) + Fl*l1*l2*m1^2*cos(the1)^2 + Fl*l1*l2*m2^2*cos(the1)^2 + Fl*l1*l2*m2^2*cos(the2)^2 + d1the1^2*l1^2*l2*m2^3*cos(the1 - the2)^2 + d1the2^2*l1*l2^2*m2^3*cos(the1 - the2)^3 - d1the1^2*l1^2*l2*m*m1^2 - d1the1^2*l1^2*l2*m*m2^2 - 3*d1the1^2*l1^2*l2*m1*m2^2 - 3*d1the1^2*l1^2*l2*m1^2*m2 + d1the1^2*l1^2*l2*m2^3*sin(the1 - the2)^2 + g*l1*l2*m1^3*cos(the1)^3 + g*l1*l2*m2^3*cos(the1)^3 + Fl*l1*l2*m2^2*cos(the1 - the2)^2 + bl*d1l1*l1*l2*m1^2 + bl*d1l1*l1*l2*m2^2 - bl*d1l1*l1*l2*m1^2*cos(the1)^2 - bl*d1l1*l1*l2*m2^2*cos(the1)^2 - bl*d1l1*l1*l2*m2^2*cos(the2)^2 + d1the1^2*l1^2*l2*m*m2^2*sin(the1 - the2)^2 + 2*d1the1^2*l1^2*l2*m1*m2^2*sin(the1 - the2)^2 + d1the1^2*l1^2*l2*m1^2*m2*sin(the1 - the2)^2 + 3*g*l1*l2*m1*m2^2*cos(the1)^3 + 3*g*l1*l2*m1^2*m2*cos(the1)^3 + bc*d1the1*l2*m1^2*cos(the1)*sin(the1) + bc*d1the1*l2*m2^2*cos(the1)*sin(the1) + bc*d1the2*l1*m1^2*cos(the2)*sin(the1) + bc*d1the2*l1*m2^2*cos(the2)*sin(the1) - bl*d1l1*l1*l2*m2^2*cos(the1 - the2)^2 - Fx*l1*l2*m2^2*sin(the1 - the2)*cos(the2) + 2*Fx*l1*l2*m1*m2*sin(the1) + d1the2^2*l1*l2^2*m2^3*cos(the1 - the2)*cos(the1)^2 + d1the2^2*l1*l2^2*m2^3*cos(the1 - the2)*cos(the2)^2 - g*l1*l2*m2^3*sin(the1 - the2)*sin(the2) + g*l1*l2*m2^3*cos(the1)*cos(the2)^2 + bc*d1the1*l2*m2^2*cos(the1 - the2)*sin(the1 - the2) - bc*d1the2*l1*m*m1*sin(the1 - the2) - bc*d1the2*l1*m*m2*sin(the1 - the2) - 2*bc*d1the2*l1*m1*m2*sin(the1 - the2) + g*l1*l2*m1^3*cos(the1)*sin(the1)^2 + g*l1*l2*m2^3*cos(the1)*sin(the1)^2 + 2*Fl*l1*l2*m1*m2*cos(the1)^2 + Fl*l1*l2*m1*m2*cos(the2)^2 - Fx*l1*l2*m2^2*cos(the1 - the2)^2*sin(the1) - d1the2^2*l1*l2^2*m*m2^2*cos(the1 - the2) - 2*d1the2^2*l1*l2^2*m1*m2^2*cos(the1 - the2) - d1the2^2*l1*l2^2*m1^2*m2*cos(the1 - the2) - 2*d1the1^2*l1^2*l2*m*m1*m2 + d1the2^2*l1*l2^2*m2^3*cos(the1 - the2)*sin(the1 - the2)^2 + g*l1*l2*m2^3*cos(the1 - the2)^2*cos(the1) - g*l1*l2*m*m1^2*cos(the1) - g*l1*l2*m*m2^2*cos(the1) - 3*g*l1*l2*m1*m2^2*cos(the1) - 3*g*l1*l2*m1^2*m2*cos(the1) + bc*d1the2*l1*m1^2*sin(the1 - the2)*cos(the1)^2 + bc*d1the2*l1*m2^2*sin(the1 - the2)*cos(the1)^2 - bx*d1x*l1*l2*m1^2*sin(the1) - bx*d1x*l1*l2*m2^2*sin(the1) + Fl*l1*l2*m*m2*cos(the1 - the2)^2 + Fl*l1*l2*m1*m2*cos(the1 - the2)^2 + 3*d1the1^2*l1^2*l2*m1*m2^2*cos(the1)^2 + 3*d1the1^2*l1^2*l2*m1^2*m2*cos(the1)^2 + 2*d1the1^2*l1^2*l2*m1*m2^2*cos(the2)^2 + d1the1^2*l1^2*l2*m1^2*m2*cos(the2)^2 + bl*d1l1*l1*l2*m*m1 + bl*d1l1*l1*l2*m*m2 + 2*bl*d1l1*l1*l2*m1*m2 - d1the1^2*l1^2*l2*m2^3*cos(the1 - the2)^2*sin(the1)^2 - d1the1^2*l1^2*l2*m2^3*sin(the1 - the2)^2*cos(the1)^2 + 3*d1the1^2*l1^2*l2*m1*m2^2*sin(the1)^2 + 3*d1the1^2*l1^2*l2*m1^2*m2*sin(the1)^2 + d1the2^2*l1*l2^2*m2^3*sin(the1)*sin(the2) + d1the1^2*l1^2*l2*m*m2^2*cos(the1 - the2)^2 + 2*d1the1^2*l1^2*l2*m1*m2^2*cos(the1 - the2)^2 + d1the1^2*l1^2*l2*m1^2*m2*cos(the1 - the2)^2 + d1the2^2*l1*l2^2*m*m2^2*cos(the1 - the2)^3 + d1the2^2*l1*l2^2*m1*m2^2*cos(the1 - the2)^3 - 2*d1the1^2*l1^2*l2*m2^3*sin(the1 - the2)*cos(the2)*sin(the1) + d1the2^2*l1*l2^2*m2^3*sin(the1 - the2)*cos(the1)*sin(the1) - d1the2^2*l1*l2^2*m2^3*sin(the1 - the2)*cos(the2)*sin(the2) - 2*Fl*l1*l2*m2^2*cos(the1 - the2)*cos(the1)*cos(the2) + d1the1^2*l1^2*l2*m*m1*m2*cos(the1 - the2)^2 - 2*bl*d1l1*l1*l2*m1*m2*cos(the1)^2 - bl*d1l1*l1*l2*m1*m2*cos(the2)^2 + g*l1*l2*m2^3*cos(the2)*sin(the1)*sin(the2) + d1the2^2*l1*l2^2*m*m2^2*cos(the1 - the2)*sin(the1 - the2)^2 + d1the2^2*l1*l2^2*m1*m2^2*cos(the1 - the2)*sin(the1 - the2)^2 + g*l1*l2*m*m2^2*cos(the1 - the2)^2*cos(the1) + 2*g*l1*l2*m1*m2^2*cos(the1 - the2)^2*cos(the1) + g*l1*l2*m1^2*m2*cos(the1 - the2)^2*cos(the1) + d1the1^2*l1^2*l2*m*m1*m2*sin(the1 - the2)^2 + bx*d1x*l1*l2*m2^2*cos(the1 - the2)^2*sin(the1) - bc*d1the2*l1*m1^2*cos(the1 - the2)*cos(the1)*sin(the1) - bc*d1the2*l1*m2^2*cos(the1 - the2)*cos(the1)*sin(the1) - bc*d1the1*l2*m2^2*cos(the1 - the2)*cos(the2)*sin(the1) - bc*d1the1*l2*m2^2*sin(the1 - the2)*cos(the1)*cos(the2) + 2*bc*d1the1*l2*m1*m2*cos(the1)*sin(the1) + 2*bc*d1the2*l1*m1*m2*cos(the2)*sin(the1) - 2*d1the2^2*l1*l2^2*m2^3*cos(the1 - the2)^2*cos(the1)*cos(the2) - bl*d1l1*l1*l2*m*m2*cos(the1 - the2)^2 - bl*d1l1*l1*l2*m1*m2*cos(the1 - the2)^2 - 2*d1the1^2*l1^2*l2*m1*m2^2*cos(the1 - the2)^2*sin(the1)^2 - 2*d1the1^2*l1^2*l2*m1*m2^2*sin(the1 - the2)^2*cos(the1)^2 - d1the1^2*l1^2*l2*m1^2*m2*cos(the1 - the2)^2*sin(the1)^2 - d1the1^2*l1^2*l2*m1^2*m2*sin(the1 - the2)^2*cos(the1)^2 + Fx*l1*l2*m2^2*cos(the1 - the2)*sin(the1 - the2)*cos(the1) - Fx*l1*l2*m1*m2*sin(the1 - the2)*cos(the2) - d1the2^2*l1*l2^2*m2^3*sin(the1 - the2)^2*cos(the1)*cos(the2) - d1the2^2*l1*l2^2*m2^3*cos(the1 - the2)^2*sin(the1)*sin(the2) + 2*d1the2^2*l1*l2^2*m1*m2^2*sin(the1)*sin(the2) + d1the2^2*l1*l2^2*m1^2*m2*sin(the1)*sin(the2) + g*l1*l2*m2^3*cos(the1 - the2)*sin(the1 - the2)*sin(the1) - 2*g*l1*l2*m2^3*cos(the1 - the2)*cos(the1)^2*cos(the2) + bc*d1the1*l2*m*m2*cos(the1 - the2)*sin(the1 - the2) + bc*d1the1*l2*m1*m2*cos(the1 - the2)*sin(the1 - the2) - g*l1*l2*m2^3*cos(the1 - the2)*cos(the2)*sin(the1)^2 + g*l1*l2*m2^3*sin(the1 - the2)*cos(the1)^2*sin(the2) - Fx*l1*l2*m1*m2*cos(the1 - the2)^2*sin(the1) - d1the2^2*l1*l2^2*m*m1*m2*cos(the1 - the2) - 2*g*l1*l2*m*m1*m2*cos(the1) + bx*d1x*l1*l2*m2^2*sin(the1 - the2)*cos(the2) + 2*bc*d1the2*l1*m1*m2*sin(the1 - the2)*cos(the1)^2 - 2*bx*d1x*l1*l2*m1*m2*sin(the1) + 2*d1the2^2*l1*l2^2*m1*m2^2*cos(the1 - the2)*cos(the1)^2 + d1the2^2*l1*l2^2*m1^2*m2*cos(the1 - the2)*cos(the1)^2 + d1the2^2*l1*l2^2*m1*m2^2*cos(the1 - the2)*cos(the2)^2 - g*l1*l2*m*m2^2*sin(the1 - the2)*sin(the2) - 2*g*l1*l2*m1*m2^2*sin(the1 - the2)*sin(the2) - g*l1*l2*m1^2*m2*sin(the1 - the2)*sin(the2) - 2*d1the1^2*l1^2*l2*m2^3*cos(the1 - the2)*cos(the1)*cos(the2) + 2*g*l1*l2*m1*m2^2*cos(the1)*cos(the2)^2 + g*l1*l2*m1^2*m2*cos(the1)*cos(the2)^2 + 3*g*l1*l2*m1*m2^2*cos(the1)*sin(the1)^2 + 3*g*l1*l2*m1^2*m2*cos(the1)*sin(the1)^2 - 2*g*l1*l2*m1*m2^2*cos(the1 - the2)*cos(the2)*sin(the1)^2 - g*l1*l2*m1^2*m2*cos(the1 - the2)*cos(the2)*sin(the1)^2 + 2*d1the1^2*l1^2*l2*m2^3*cos(the1 - the2)*sin(the1 - the2)*cos(the1)*sin(the1) + d1the2^2*l1*l2^2*m2^3*cos(the1 - the2)*sin(the1 - the2)*cos(the1)*sin(the2) - d1the2^2*l1*l2^2*m2^3*cos(the1 - the2)*sin(the1 - the2)*cos(the2)*sin(the1) + 2*g*l1*l2*m1*m2^2*sin(the1 - the2)*cos(the1)^2*sin(the2) + g*l1*l2*m1^2*m2*sin(the1 - the2)*cos(the1)^2*sin(the2) - 2*Fl*l1*l2*m1*m2*cos(the1 - the2)*cos(the1)*cos(the2) - g*l1*l2*m2^3*cos(the1 - the2)*cos(the1)*sin(the1)*sin(the2) - g*l1*l2*m2^3*sin(the1 - the2)*cos(the1)*cos(the2)*sin(the1) + g*l1*l2*m*m1*m2*cos(the1 - the2)^2*cos(the1) + bx*d1x*l1*l2*m1*m2*cos(the1 - the2)^2*sin(the1) - 2*bc*d1the2*l1*m1*m2*cos(the1 - the2)*cos(the1)*sin(the1) - bc*d1the1*l2*m1*m2*cos(the1 - the2)*cos(the2)*sin(the1) - bc*d1the1*l2*m1*m2*sin(the1 - the2)*cos(the1)*cos(the2) - 4*d1the1^2*l1^2*l2*m1*m2^2*cos(the1 - the2)*cos(the1)*cos(the2) - 2*d1the1^2*l1^2*l2*m1^2*m2*cos(the1 - the2)*cos(the1)*cos(the2) + Fx*l1*l2*m1*m2*cos(the1 - the2)*sin(the1 - the2)*cos(the1) - 4*d1the1^2*l1^2*l2*m1*m2^2*sin(the1 - the2)*cos(the2)*sin(the1) - 2*d1the1^2*l1^2*l2*m1^2*m2*sin(the1 - the2)*cos(the2)*sin(the1) + 2*d1the2^2*l1*l2^2*m1*m2^2*sin(the1 - the2)*cos(the1)*sin(the1) + d1the2^2*l1*l2^2*m1^2*m2*sin(the1 - the2)*cos(the1)*sin(the1) - d1the2^2*l1*l2^2*m1*m2^2*sin(the1 - the2)*cos(the2)*sin(the2) + 2*g*l1*l2*m1*m2^2*cos(the2)*sin(the1)*sin(the2) + g*l1*l2*m1^2*m2*cos(the2)*sin(the1)*sin(the2) + 2*bl*d1l1*l1*l2*m2^2*cos(the1 - the2)*cos(the1)*cos(the2) - 2*d1the2^2*l1*l2^2*m1*m2^2*cos(the1 - the2)^2*cos(the1)*cos(the2) - d1the2^2*l1*l2^2*m1*m2^2*sin(the1 - the2)^2*cos(the1)*cos(the2) - bx*d1x*l1*l2*m2^2*cos(the1 - the2)*sin(the1 - the2)*cos(the1) + bx*d1x*l1*l2*m1*m2*sin(the1 - the2)*cos(the2) - d1the2^2*l1*l2^2*m1*m2^2*cos(the1 - the2)^2*sin(the1)*sin(the2) + g*l1*l2*m*m2^2*cos(the1 - the2)*sin(the1 - the2)*sin(the1) + 2*g*l1*l2*m1*m2^2*cos(the1 - the2)*sin(the1 - the2)*sin(the1) + g*l1*l2*m1^2*m2*cos(the1 - the2)*sin(the1 - the2)*sin(the1) - g*l1*l2*m*m1*m2*sin(the1 - the2)*sin(the2) - 4*g*l1*l2*m1*m2^2*cos(the1 - the2)*cos(the1)^2*cos(the2) - 2*g*l1*l2*m1^2*m2*cos(the1 - the2)*cos(the1)^2*cos(the2) + 4*d1the1^2*l1^2*l2*m1*m2^2*cos(the1 - the2)*sin(the1 - the2)*cos(the1)*sin(the1) + 2*d1the1^2*l1^2*l2*m1^2*m2*cos(the1 - the2)*sin(the1 - the2)*cos(the1)*sin(the1) + d1the2^2*l1*l2^2*m1*m2^2*cos(the1 - the2)*sin(the1 - the2)*cos(the1)*sin(the2) - d1the2^2*l1*l2^2*m1*m2^2*cos(the1 - the2)*sin(the1 - the2)*cos(the2)*sin(the1) - 2*g*l1*l2*m1*m2^2*cos(the1 - the2)*cos(the1)*sin(the1)*sin(the2) - 2*g*l1*l2*m1*m2^2*sin(the1 - the2)*cos(the1)*cos(the2)*sin(the1) - g*l1*l2*m1^2*m2*cos(the1 - the2)*cos(the1)*sin(the1)*sin(the2) - g*l1*l2*m1^2*m2*sin(the1 - the2)*cos(the1)*cos(the2)*sin(the1) + 2*bl*d1l1*l1*l2*m1*m2*cos(the1 - the2)*cos(the1)*cos(the2) - bx*d1x*l1*l2*m1*m2*cos(the1 - the2)*sin(the1 - the2)*cos(the1) + g*l1*l2*m*m1*m2*cos(the1 - the2)*sin(the1 - the2)*sin(the1))/(l1*l2*(m1 + m2)*(m1^2*cos(the1)^2 - m*m2 - 2*m1*m2 - m*m1 + m2^2*cos(the1)^2 + m2^2*cos(the2)^2 + m1^2*sin(the1)^2 + m2^2*sin(the1)^2 + m2^2*cos(the1 - the2)^2 + m2^2*sin(the1 - the2)^2 - m1^2 - m2^2 + 2*m1*m2*cos(the1)^2 + m1*m2*cos(the2)^2 + 2*m1*m2*sin(the1)^2 + m*m2*cos(the1 - the2)^2 + m1*m2*cos(the1 - the2)^2 + m*m2*sin(the1 - the2)^2 + m1*m2*sin(the1 - the2)^2 - m2^2*cos(the1 - the2)^2*sin(the1)^2 - m2^2*sin(the1 - the2)^2*cos(the1)^2 - 2*m2^2*sin(the1 - the2)*cos(the2)*sin(the1) - 2*m2^2*cos(the1 - the2)*cos(the1)*cos(the2) - m1*m2*cos(the1 - the2)^2*sin(the1)^2 - m1*m2*sin(the1 - the2)^2*cos(the1)^2 + 2*m2^2*cos(the1 - the2)*sin(the1 - the2)*cos(the1)*sin(the1) - 2*m1*m2*sin(the1 - the2)*cos(the2)*sin(the1) - 2*m1*m2*cos(the1 - the2)*cos(the1)*cos(the2) + 2*m1*m2*cos(the1 - the2)*sin(the1 - the2)*cos(the1)*sin(the1)));
 
 dx5=d1the1;

 dx6 = -(bc*d1the2*l1*m1^2*cos(the1 - the2) - bc*d1the1*l2*m2^2 - Fx*l1*l2*m1^2*cos(the1) - Fx*l1*l2*m2^2*cos(the1) - d1the2^2*l1*l2^2*m2^3*sin(the1 - the2) - g*l1*l2*m1^3*sin(the1) - g*l1*l2*m2^3*sin(the1) - bc*d1the1*l2*m1^2 + bc*d1the2*l1*m2^2*cos(the1 - the2) - bc*d1the1*l2*m*m1 - bc*d1the1*l2*m*m2 - 2*bc*d1the1*l2*m1*m2 + bc*d1the1*l2*m2^2*cos(the2)^2 + d1the2^2*l1*l2^2*m2^3*sin(the1 - the2)^3 + bc*d1the1*l2*m1^2*sin(the1)^2 + bc*d1the1*l2*m2^2*sin(the1)^2 + g*l1*l2*m1^3*sin(the1)^3 + g*l1*l2*m2^3*sin(the1)^3 - 2*d1l1*d1the1*l1*l2*m1^3 - 2*d1l1*d1the1*l1*l2*m2^3 + bc*d1the1*l2*m2^2*sin(the1 - the2)^2 + 2*d1l1*d1the1*l1*l2*m1^3*cos(the1)^2 + 2*d1l1*d1the1*l1*l2*m2^3*cos(the1)^2 + 2*d1l1*d1the1*l1*l2*m2^3*cos(the2)^2 + Fl*l1*l2*m1^2*cos(the1)*sin(the1) + Fl*l1*l2*m2^2*cos(the1)*sin(the1) - bc*d1the2*l1*m1^2*cos(the1)*cos(the2) - bc*d1the2*l1*m2^2*cos(the1)*cos(the2) + d1the2^2*l1*l2^2*m*m2^2*sin(the1 - the2)^3 + d1the2^2*l1*l2^2*m1*m2^2*sin(the1 - the2)^3 + 2*d1l1*d1the1*l1*l2*m1^3*sin(the1)^2 + 2*d1l1*d1the1*l1*l2*m2^3*sin(the1)^2 + 3*g*l1*l2*m1*m2^2*sin(the1)^3 + 3*g*l1*l2*m1^2*m2*sin(the1)^3 + Fx*l1*l2*m2^2*cos(the1 - the2)*cos(the2) - 2*Fx*l1*l2*m1*m2*cos(the1) + 2*d1l1*d1the1*l1*l2*m2^3*cos(the1 - the2)^2 - 2*d1l1*d1the1*l1*l2*m*m1^2 - 2*d1l1*d1the1*l1*l2*m*m2^2 - 6*d1l1*d1the1*l1*l2*m1*m2^2 - 6*d1l1*d1the1*l1*l2*m1^2*m2 + 2*d1l1*d1the1*l1*l2*m2^3*sin(the1 - the2)^2 + g*l1*l2*m2^3*cos(the1 - the2)*sin(the2) + Fl*l1*l2*m2^2*cos(the1 - the2)*sin(the1 - the2) + bc*d1the2*l1*m*m1*cos(the1 - the2) + bc*d1the2*l1*m*m2*cos(the1 - the2) + 2*bc*d1the2*l1*m1*m2*cos(the1 - the2) + d1the2^2*l1*l2^2*m2^3*sin(the1 - the2)*cos(the2)^2 + d1the2^2*l1*l2^2*m2^3*sin(the1 - the2)*sin(the1)^2 + g*l1*l2*m1^3*cos(the1)^2*sin(the1) + g*l1*l2*m2^3*cos(the1)^2*sin(the1) + g*l1*l2*m2^3*cos(the2)^2*sin(the1) + Fx*l1*l2*m2^2*sin(the1 - the2)^2*cos(the1) + bx*d1x*l1*l2*m1^2*cos(the1) + bx*d1x*l1*l2*m2^2*cos(the1) + bc*d1the1*l2*m1*m2*cos(the2)^2 + d1the2^2*l1*l2^2*m2^3*cos(the1 - the2)^2*sin(the1 - the2) - d1the2^2*l1*l2^2*m*m2^2*sin(the1 - the2) - 2*d1the2^2*l1*l2^2*m1*m2^2*sin(the1 - the2) - d1the2^2*l1*l2^2*m1^2*m2*sin(the1 - the2) - bc*d1the2*l1*m1^2*cos(the1 - the2)*sin(the1)^2 - bc*d1the2*l1*m2^2*cos(the1 - the2)*sin(the1)^2 + 2*bc*d1the1*l2*m1*m2*sin(the1)^2 - g*l1*l2*m*m1^2*sin(the1) - g*l1*l2*m*m2^2*sin(the1) - 3*g*l1*l2*m1*m2^2*sin(the1) - 3*g*l1*l2*m1^2*m2*sin(the1) + g*l1*l2*m2^3*sin(the1 - the2)^2*sin(the1) + bc*d1the1*l2*m*m2*sin(the1 - the2)^2 + bc*d1the1*l2*m1*m2*sin(the1 - the2)^2 - d1the2^2*l1*l2^2*m2^3*cos(the1)*sin(the2) - g*l1*l2*m2^3*cos(the1)*cos(the2)*sin(the2) - Fl*l1*l2*m2^2*cos(the1 - the2)*cos(the2)*sin(the1) - Fl*l1*l2*m2^2*sin(the1 - the2)*cos(the1)*cos(the2) + 2*Fl*l1*l2*m1*m2*cos(the1)*sin(the1) + d1the2^2*l1*l2^2*m*m2^2*cos(the1 - the2)^2*sin(the1 - the2) + d1the2^2*l1*l2^2*m1*m2^2*cos(the1 - the2)^2*sin(the1 - the2) - 2*bc*d1the2*l1*m1*m2*cos(the1)*cos(the2) - bx*d1x*l1*l2*m2^2*sin(the1 - the2)^2*cos(the1) + bc*d1the2*l1*m1^2*sin(the1 - the2)*cos(the1)*sin(the1) + bc*d1the2*l1*m2^2*sin(the1 - the2)*cos(the1)*sin(the1) - 2*bc*d1the1*l2*m2^2*sin(the1 - the2)*cos(the2)*sin(the1) + g*l1*l2*m*m2^2*sin(the1 - the2)^2*sin(the1) + 2*g*l1*l2*m1*m2^2*sin(the1 - the2)^2*sin(the1) + g*l1*l2*m1^2*m2*sin(the1 - the2)^2*sin(the1) + Fx*l1*l2*m1*m2*cos(the1 - the2)*cos(the2) - 4*d1l1*d1the1*l1*l2*m*m1*m2 - d1the2^2*l1*l2^2*m2^3*cos(the1 - the2)^2*cos(the2)*sin(the1) - 2*d1the2^2*l1*l2^2*m1*m2^2*cos(the1)*sin(the2) - d1the2^2*l1*l2^2*m1^2*m2*cos(the1)*sin(the2) - Fx*l1*l2*m2^2*cos(the1 - the2)*sin(the1 - the2)*sin(the1) + d1the2^2*l1*l2^2*m2^3*sin(the1 - the2)^2*cos(the1)*sin(the2) - 2*d1the2^2*l1*l2^2*m2^3*sin(the1 - the2)^2*cos(the2)*sin(the1) + g*l1*l2*m2^3*cos(the1 - the2)*sin(the1 - the2)*cos(the1) + 6*d1l1*d1the1*l1*l2*m1*m2^2*cos(the1)^2 + 6*d1l1*d1the1*l1*l2*m1^2*m2*cos(the1)^2 + 4*d1l1*d1the1*l1*l2*m1*m2^2*cos(the2)^2 + 2*d1l1*d1the1*l1*l2*m1^2*m2*cos(the2)^2 - 2*d1l1*d1the1*l1*l2*m2^3*cos(the1 - the2)^2*sin(the1)^2 - 2*d1l1*d1the1*l1*l2*m2^3*sin(the1 - the2)^2*cos(the1)^2 + Fl*l1*l2*m*m2*cos(the1 - the2)*sin(the1 - the2) + Fl*l1*l2*m1*m2*cos(the1 - the2)*sin(the1 - the2) + 6*d1l1*d1the1*l1*l2*m1*m2^2*sin(the1)^2 + 6*d1l1*d1the1*l1*l2*m1^2*m2*sin(the1)^2 - bl*d1l1*l1*l2*m1^2*cos(the1)*sin(the1) - bl*d1l1*l1*l2*m2^2*cos(the1)*sin(the1) - g*l1*l2*m2^3*sin(the1 - the2)*cos(the1)^2*cos(the2) + 2*d1l1*d1the1*l1*l2*m*m2^2*cos(the1 - the2)^2 + 4*d1l1*d1the1*l1*l2*m1*m2^2*cos(the1 - the2)^2 + 2*d1l1*d1the1*l1*l2*m1^2*m2*cos(the1 - the2)^2 - g*l1*l2*m2^3*cos(the1 - the2)*sin(the1)^2*sin(the2) - 2*g*l1*l2*m2^3*sin(the1 - the2)*cos(the2)*sin(the1)^2 + Fx*l1*l2*m1*m2*sin(the1 - the2)^2*cos(the1) - bx*d1x*l1*l2*m2^2*cos(the1 - the2)*cos(the2) + 2*bx*d1x*l1*l2*m1*m2*cos(the1) + 2*d1l1*d1the1*l1*l2*m*m2^2*sin(the1 - the2)^2 + 4*d1l1*d1the1*l1*l2*m1*m2^2*sin(the1 - the2)^2 + 2*d1l1*d1the1*l1*l2*m1^2*m2*sin(the1 - the2)^2 - d1the2^2*l1*l2^2*m*m1*m2*sin(the1 - the2) - 2*bc*d1the2*l1*m1*m2*cos(the1 - the2)*sin(the1)^2 + g*l1*l2*m*m2^2*cos(the1 - the2)*sin(the2) + 2*g*l1*l2*m1*m2^2*cos(the1 - the2)*sin(the2) + g*l1*l2*m1^2*m2*cos(the1 - the2)*sin(the2) - 2*g*l1*l2*m*m1*m2*sin(the1) + d1the2^2*l1*l2^2*m1*m2^2*sin(the1 - the2)*cos(the2)^2 - bl*d1l1*l1*l2*m2^2*cos(the1 - the2)*sin(the1 - the2) + d1the2^2*l1*l2^2*m2^3*cos(the1 - the2)*cos(the1)*sin(the1) + d1the2^2*l1*l2^2*m2^3*cos(the1 - the2)*cos(the2)*sin(the2) + 2*d1the2^2*l1*l2^2*m1*m2^2*sin(the1 - the2)*sin(the1)^2 + d1the2^2*l1*l2^2*m1^2*m2*sin(the1 - the2)*sin(the1)^2 + 3*g*l1*l2*m1*m2^2*cos(the1)^2*sin(the1) + 3*g*l1*l2*m1^2*m2*cos(the1)^2*sin(the1) + 2*g*l1*l2*m1*m2^2*cos(the2)^2*sin(the1) + g*l1*l2*m1^2*m2*cos(the2)^2*sin(the1) - 2*g*l1*l2*m1*m2^2*sin(the1 - the2)*cos(the1)^2*cos(the2) - g*l1*l2*m1^2*m2*sin(the1 - the2)*cos(the1)^2*cos(the2) - g*l1*l2*m2^3*cos(the1 - the2)*cos(the1)*cos(the2)*sin(the1) - 2*g*l1*l2*m1*m2^2*cos(the1 - the2)*sin(the1)^2*sin(the2) - 4*g*l1*l2*m1*m2^2*sin(the1 - the2)*cos(the2)*sin(the1)^2 - g*l1*l2*m1^2*m2*cos(the1 - the2)*sin(the1)^2*sin(the2) - 2*g*l1*l2*m1^2*m2*sin(the1 - the2)*cos(the2)*sin(the1)^2 - d1the2^2*l1*l2^2*m2^3*cos(the1 - the2)*sin(the1 - the2)*sin(the1)*sin(the2) - Fl*l1*l2*m1*m2*cos(the1 - the2)*cos(the2)*sin(the1) - Fl*l1*l2*m1*m2*sin(the1 - the2)*cos(the1)*cos(the2) - bx*d1x*l1*l2*m1*m2*sin(the1 - the2)^2*cos(the1) + g*l1*l2*m2^3*sin(the1 - the2)*cos(the1)*sin(the1)*sin(the2) + 2*bc*d1the2*l1*m1*m2*sin(the1 - the2)*cos(the1)*sin(the1) - 2*bc*d1the1*l2*m1*m2*sin(the1 - the2)*cos(the2)*sin(the1) + g*l1*l2*m*m1*m2*sin(the1 - the2)^2*sin(the1) + 2*d1the2^2*l1*l2^2*m1*m2^2*cos(the1 - the2)*cos(the1)*sin(the1) + d1the2^2*l1*l2^2*m1^2*m2*cos(the1 - the2)*cos(the1)*sin(the1) + d1the2^2*l1*l2^2*m1*m2^2*cos(the1 - the2)*cos(the2)*sin(the2) - Fx*l1*l2*m1*m2*cos(the1 - the2)*sin(the1 - the2)*sin(the1) - 2*g*l1*l2*m1*m2^2*cos(the1)*cos(the2)*sin(the2) - g*l1*l2*m1^2*m2*cos(the1)*cos(the2)*sin(the2) - 4*d1l1*d1the1*l1*l2*m2^3*cos(the1 - the2)*cos(the1)*cos(the2) + bl*d1l1*l1*l2*m2^2*cos(the1 - the2)*cos(the2)*sin(the1) + bl*d1l1*l1*l2*m2^2*sin(the1 - the2)*cos(the1)*cos(the2) - 2*bl*d1l1*l1*l2*m1*m2*cos(the1)*sin(the1) - 4*d1l1*d1the1*l1*l2*m2^3*sin(the1 - the2)*cos(the2)*sin(the1) + 2*d1l1*d1the1*l1*l2*m*m1*m2*cos(the1 - the2)^2 - bx*d1x*l1*l2*m1*m2*cos(the1 - the2)*cos(the2) - d1the2^2*l1*l2^2*m1*m2^2*cos(the1 - the2)^2*cos(the2)*sin(the1) + 2*d1l1*d1the1*l1*l2*m*m1*m2*sin(the1 - the2)^2 + d1the2^2*l1*l2^2*m1*m2^2*sin(the1 - the2)^2*cos(the1)*sin(the2) - 2*d1the2^2*l1*l2^2*m1*m2^2*sin(the1 - the2)^2*cos(the2)*sin(the1) + g*l1*l2*m*m2^2*cos(the1 - the2)*sin(the1 - the2)*cos(the1) + 2*g*l1*l2*m1*m2^2*cos(the1 - the2)*sin(the1 - the2)*cos(the1) + g*l1*l2*m1^2*m2*cos(the1 - the2)*sin(the1 - the2)*cos(the1) + g*l1*l2*m*m1*m2*cos(the1 - the2)*sin(the2) + bx*d1x*l1*l2*m2^2*cos(the1 - the2)*sin(the1 - the2)*sin(the1) - 4*d1l1*d1the1*l1*l2*m1*m2^2*cos(the1 - the2)^2*sin(the1)^2 - 4*d1l1*d1the1*l1*l2*m1*m2^2*sin(the1 - the2)^2*cos(the1)^2 - 2*d1l1*d1the1*l1*l2*m1^2*m2*cos(the1 - the2)^2*sin(the1)^2 - 2*d1l1*d1the1*l1*l2*m1^2*m2*sin(the1 - the2)^2*cos(the1)^2 - d1the2^2*l1*l2^2*m2^3*cos(the1 - the2)*sin(the1 - the2)*cos(the1)*cos(the2) - bl*d1l1*l1*l2*m*m2*cos(the1 - the2)*sin(the1 - the2) - bl*d1l1*l1*l2*m1*m2*cos(the1 - the2)*sin(the1 - the2) - 8*d1l1*d1the1*l1*l2*m1*m2^2*sin(the1 - the2)*cos(the2)*sin(the1) - 4*d1l1*d1the1*l1*l2*m1^2*m2*sin(the1 - the2)*cos(the2)*sin(the1) - d1the2^2*l1*l2^2*m1*m2^2*cos(the1 - the2)*sin(the1 - the2)*cos(the1)*cos(the2) - 2*g*l1*l2*m1*m2^2*cos(the1 - the2)*cos(the1)*cos(the2)*sin(the1) - g*l1*l2*m1^2*m2*cos(the1 - the2)*cos(the1)*cos(the2)*sin(the1) - d1the2^2*l1*l2^2*m1*m2^2*cos(the1 - the2)*sin(the1 - the2)*sin(the1)*sin(the2) + 2*g*l1*l2*m1*m2^2*sin(the1 - the2)*cos(the1)*sin(the1)*sin(the2) + g*l1*l2*m1^2*m2*sin(the1 - the2)*cos(the1)*sin(the1)*sin(the2) + bl*d1l1*l1*l2*m1*m2*cos(the1 - the2)*cos(the2)*sin(the1) + bl*d1l1*l1*l2*m1*m2*sin(the1 - the2)*cos(the1)*cos(the2) + 4*d1l1*d1the1*l1*l2*m2^3*cos(the1 - the2)*sin(the1 - the2)*cos(the1)*sin(the1) + g*l1*l2*m*m1*m2*cos(the1 - the2)*sin(the1 - the2)*cos(the1) + bx*d1x*l1*l2*m1*m2*cos(the1 - the2)*sin(the1 - the2)*sin(the1) - 8*d1l1*d1the1*l1*l2*m1*m2^2*cos(the1 - the2)*cos(the1)*cos(the2) - 4*d1l1*d1the1*l1*l2*m1^2*m2*cos(the1 - the2)*cos(the1)*cos(the2) + 8*d1l1*d1the1*l1*l2*m1*m2^2*cos(the1 - the2)*sin(the1 - the2)*cos(the1)*sin(the1) + 4*d1l1*d1the1*l1*l2*m1^2*m2*cos(the1 - the2)*sin(the1 - the2)*cos(the1)*sin(the1))/(l1^2*l2*(m1 + m2)*(m1^2*cos(the1)^2 - m*m2 - 2*m1*m2 - m*m1 + m2^2*cos(the1)^2 + m2^2*cos(the2)^2 + m1^2*sin(the1)^2 + m2^2*sin(the1)^2 + m2^2*cos(the1 - the2)^2 + m2^2*sin(the1 - the2)^2 - m1^2 - m2^2 + 2*m1*m2*cos(the1)^2 + m1*m2*cos(the2)^2 + 2*m1*m2*sin(the1)^2 + m*m2*cos(the1 - the2)^2 + m1*m2*cos(the1 - the2)^2 + m*m2*sin(the1 - the2)^2 + m1*m2*sin(the1 - the2)^2 - m2^2*cos(the1 - the2)^2*sin(the1)^2 - m2^2*sin(the1 - the2)^2*cos(the1)^2 - 2*m2^2*sin(the1 - the2)*cos(the2)*sin(the1) - 2*m2^2*cos(the1 - the2)*cos(the1)*cos(the2) - m1*m2*cos(the1 - the2)^2*sin(the1)^2 - m1*m2*sin(the1 - the2)^2*cos(the1)^2 + 2*m2^2*cos(the1 - the2)*sin(the1 - the2)*cos(the1)*sin(the1) - 2*m1*m2*sin(the1 - the2)*cos(the2)*sin(the1) - 2*m1*m2*cos(the1 - the2)*cos(the1)*cos(the2) + 2*m1*m2*cos(the1 - the2)*sin(the1 - the2)*cos(the1)*sin(the1)));

 dx7=d1the2;

 dx8 = -(bc*d1the1*l2*m2^2*cos(the1 - the2) - bc*d1the2*l1*m2^2 - Fx*l1*l2*m2^2*cos(the2) - g*l1*l2*m2^3*sin(the2) - Fl*l1*l2*m2^2*sin(the1 - the2) - bc*d1the2*l1*m1^2 - bc*d1the2*l1*m*m1 - bc*d1the2*l1*m*m2 - 2*bc*d1the2*l1*m1*m2 + bc*d1the2*l1*m1^2*cos(the1)^2 + bc*d1the2*l1*m2^2*cos(the1)^2 + bc*d1the2*l1*m1^2*sin(the1)^2 + bc*d1the2*l1*m2^2*sin(the1)^2 + Fl*l1*l2*m2^2*cos(the2)*sin(the1) - bc*d1the1*l2*m2^2*cos(the1)*cos(the2) + Fx*l1*l2*m2^2*cos(the1 - the2)*cos(the1) - Fx*l1*l2*m1*m2*cos(the2) + Fx*l1*l2*m2^2*sin(the1 - the2)*sin(the1) + g*l1*l2*m2^3*cos(the1 - the2)*sin(the1) - g*l1*l2*m2^3*sin(the1 - the2)*cos(the1) - Fl*l1*l2*m*m2*sin(the1 - the2) - Fl*l1*l2*m1*m2*sin(the1 - the2) + bc*d1the1*l2*m*m2*cos(the1 - the2) + bc*d1the1*l2*m1*m2*cos(the1 - the2) + g*l1*l2*m2^3*cos(the1)^2*sin(the2) + g*l1*l2*m2^3*sin(the1)^2*sin(the2) + Fl*l1*l2*m2^2*sin(the1 - the2)*cos(the1)^2 + bx*d1x*l1*l2*m2^2*cos(the2) + 2*bc*d1the2*l1*m1*m2*cos(the1)^2 - bc*d1the1*l2*m2^2*cos(the1 - the2)*sin(the1)^2 + 2*bc*d1the2*l1*m1*m2*sin(the1)^2 - g*l1*l2*m2^3*cos(the1 - the2)*sin(the1)^3 + g*l1*l2*m2^3*sin(the1 - the2)*cos(the1)^3 - g*l1*l2*m*m2^2*sin(the2) - 2*g*l1*l2*m1*m2^2*sin(the2) - g*l1*l2*m1^2*m2*sin(the2) + bl*d1l1*l1*l2*m2^2*sin(the1 - the2) - d1the2^2*l1*l2^2*m2^3*cos(the2)*sin(the2) + 2*g*l1*l2*m1*m2^2*sin(the1)^2*sin(the2) + g*l1*l2*m1^2*m2*sin(the1)^2*sin(the2) + d1the2^2*l1*l2^2*m2^3*sin(the1 - the2)*sin(the1)*sin(the2) - Fl*l1*l2*m2^2*cos(the1 - the2)*cos(the1)*sin(the1) + Fl*l1*l2*m1*m2*cos(the2)*sin(the1) - bc*d1the1*l2*m1*m2*cos(the1)*cos(the2) - bl*d1l1*l1*l2*m2^2*sin(the1 - the2)*cos(the1)^2 - 2*g*l1*l2*m1*m2^2*cos(the1 - the2)*sin(the1)^3 + 2*g*l1*l2*m1*m2^2*sin(the1 - the2)*cos(the1)^3 - g*l1*l2*m1^2*m2*cos(the1 - the2)*sin(the1)^3 + g*l1*l2*m1^2*m2*sin(the1 - the2)*cos(the1)^3 + bc*d1the1*l2*m2^2*sin(the1 - the2)*cos(the1)*sin(the1) + Fx*l1*l2*m1*m2*cos(the1 - the2)*cos(the1) - d1the2^2*l1*l2^2*m2^3*cos(the1 - the2)^2*cos(the1)*sin(the1) - d1the2^2*l1*l2^2*m1*m2^2*cos(the2)*sin(the2) + Fx*l1*l2*m1*m2*sin(the1 - the2)*sin(the1) + d1the2^2*l1*l2^2*m2^3*sin(the1 - the2)^2*cos(the1)*sin(the1) + d1the2^2*l1*l2^2*m2^3*cos(the1 - the2)*sin(the1 - the2)*cos(the1)^2 - bl*d1l1*l1*l2*m2^2*cos(the2)*sin(the1) - d1the2^2*l1*l2^2*m2^3*cos(the1 - the2)*sin(the1 - the2)*sin(the1)^2 - g*l1*l2*m2^3*cos(the1 - the2)*cos(the1)^2*sin(the1) + g*l1*l2*m2^3*sin(the1 - the2)*cos(the1)*sin(the1)^2 + Fl*l1*l2*m1*m2*sin(the1 - the2)*cos(the1)^2 - bx*d1x*l1*l2*m2^2*cos(the1 - the2)*cos(the1) + bx*d1x*l1*l2*m1*m2*cos(the2) - bc*d1the1*l2*m1*m2*cos(the1 - the2)*sin(the1)^2 + g*l1*l2*m*m2^2*cos(the1 - the2)*sin(the1) - g*l1*l2*m*m2^2*sin(the1 - the2)*cos(the1) + 2*g*l1*l2*m1*m2^2*cos(the1 - the2)*sin(the1) - 2*g*l1*l2*m1*m2^2*sin(the1 - the2)*cos(the1) + g*l1*l2*m1^2*m2*cos(the1 - the2)*sin(the1) - g*l1*l2*m1^2*m2*sin(the1 - the2)*cos(the1) - g*l1*l2*m*m1*m2*sin(the2) - bx*d1x*l1*l2*m2^2*sin(the1 - the2)*sin(the1) + d1the2^2*l1*l2^2*m2^3*cos(the1 - the2)*cos(the1)*sin(the2) + d1the2^2*l1*l2^2*m2^3*cos(the1 - the2)*cos(the2)*sin(the1) - d1the2^2*l1*l2^2*m2^3*sin(the1 - the2)*cos(the1)*cos(the2) + bl*d1l1*l1*l2*m*m2*sin(the1 - the2) + bl*d1l1*l1*l2*m1*m2*sin(the1 - the2) + 2*g*l1*l2*m1*m2^2*cos(the1)^2*sin(the2) + g*l1*l2*m1^2*m2*cos(the1)^2*sin(the2) - d1the2^2*l1*l2^2*m1*m2^2*cos(the1 - the2)*sin(the1 - the2)*sin(the1)^2 - 2*g*l1*l2*m1*m2^2*cos(the1 - the2)*cos(the1)^2*sin(the1) - g*l1*l2*m1^2*m2*cos(the1 - the2)*cos(the1)^2*sin(the1) + 2*g*l1*l2*m1*m2^2*sin(the1 - the2)*cos(the1)*sin(the1)^2 + g*l1*l2*m1^2*m2*sin(the1 - the2)*cos(the1)*sin(the1)^2 - Fl*l1*l2*m1*m2*cos(the1 - the2)*cos(the1)*sin(the1) - bl*d1l1*l1*l2*m1*m2*sin(the1 - the2)*cos(the1)^2 + bc*d1the1*l2*m1*m2*sin(the1 - the2)*cos(the1)*sin(the1) + d1the2^2*l1*l2^2*m1*m2^2*cos(the1 - the2)*cos(the1)*sin(the2) + d1the2^2*l1*l2^2*m1*m2^2*cos(the1 - the2)*cos(the2)*sin(the1) - d1the2^2*l1*l2^2*m1*m2^2*sin(the1 - the2)*cos(the1)*cos(the2) + d1the2^2*l1*l2^2*m1*m2^2*sin(the1 - the2)*sin(the1)*sin(the2) + bl*d1l1*l1*l2*m2^2*cos(the1 - the2)*cos(the1)*sin(the1) - bl*d1l1*l1*l2*m1*m2*cos(the2)*sin(the1) - bx*d1x*l1*l2*m1*m2*cos(the1 - the2)*cos(the1) - d1the2^2*l1*l2^2*m1*m2^2*cos(the1 - the2)^2*cos(the1)*sin(the1) + d1the2^2*l1*l2^2*m1*m2^2*sin(the1 - the2)^2*cos(the1)*sin(the1) + g*l1*l2*m*m1*m2*cos(the1 - the2)*sin(the1) - g*l1*l2*m*m1*m2*sin(the1 - the2)*cos(the1) - bx*d1x*l1*l2*m1*m2*sin(the1 - the2)*sin(the1) + d1the2^2*l1*l2^2*m1*m2^2*cos(the1 - the2)*sin(the1 - the2)*cos(the1)^2 + bl*d1l1*l1*l2*m1*m2*cos(the1 - the2)*cos(the1)*sin(the1))/(l1*l2^2*m2*(m1^2*cos(the1)^2 - m*m2 - 2*m1*m2 - m*m1 + m2^2*cos(the1)^2 + m2^2*cos(the2)^2 + m1^2*sin(the1)^2 + m2^2*sin(the1)^2 + m2^2*cos(the1 - the2)^2 + m2^2*sin(the1 - the2)^2 - m1^2 - m2^2 + 2*m1*m2*cos(the1)^2 + m1*m2*cos(the2)^2 + 2*m1*m2*sin(the1)^2 + m*m2*cos(the1 - the2)^2 + m1*m2*cos(the1 - the2)^2 + m*m2*sin(the1 - the2)^2 + m1*m2*sin(the1 - the2)^2 - m2^2*cos(the1 - the2)^2*sin(the1)^2 - m2^2*sin(the1 - the2)^2*cos(the1)^2 - 2*m2^2*sin(the1 - the2)*cos(the2)*sin(the1) - 2*m2^2*cos(the1 - the2)*cos(the1)*cos(the2) - m1*m2*cos(the1 - the2)^2*sin(the1)^2 - m1*m2*sin(the1 - the2)^2*cos(the1)^2 + 2*m2^2*cos(the1 - the2)*sin(the1 - the2)*cos(the1)*sin(the1) - 2*m1*m2*sin(the1 - the2)*cos(the2)*sin(the1) - 2*m1*m2*cos(the1 - the2)*cos(the1)*cos(the2) + 2*m1*m2*cos(the1 - the2)*sin(the1 - the2)*cos(the1)*sin(the1)));
